simulink model "Proj_5_part_2"  (R2016b)
settings: Solver=ode4  StartTime=0.0  StopTime=1370  FixedStep=0.0001  RelTol=1e-3
undefined symbols (not defined in the file or in its folder): V
settings Model: Creator=apple  LastModifiedBy=apple

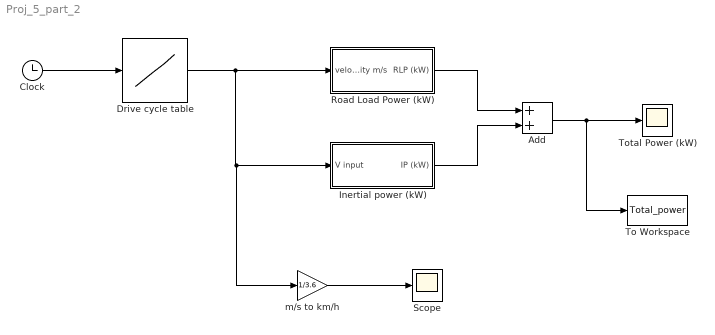
== system Proj_5_part_2 ==
  Add : Sum
  Clock : Clock
  Drive cycle table : Lookup_n-D  NumberOfTableDimensions=1  BreakpointsForDimension1=t  Table=V  InternalRulePriority=Speed  RndMeth=Simplest  InputSameDT=on
  Inertial power (kW) : Subsystem  TreatAsAtomicUnit=on
  Road Load Power (kW) : Subsystem  TreatAsAtomicUnit=on
  Scope : Scope
  To Workspace : ToWorkspace  VariableName=Total_power  SaveFormat=Timeseries  SampleTime=-1
  Total Power (kW) : Scope
  m/s to km/h : Gain  Gain=1/3.6
  wires:
  Clock/1 -> Drive cycle table/1
  Drive cycle table/1 -> m/s to km/h/1, Inertial power (kW)/1(V input), Road Load Power (kW)/1("velocity m/s ")
  Road Load Power (kW)/1(RLP (kW)) -> Add/1
  Inertial power (kW)/1(IP (kW)) -> Add/2
  Add/1 -> To Workspace/1, Total Power (kW)/1
  m/s to km/h/1 -> Scope/1

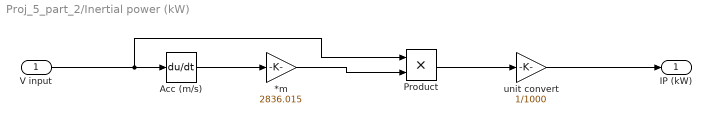
== system Proj_5_part_2/Inertial power (kW) ==
  V input : Inport
  *m : Gain  Gain=2836.015
  Acc (m/s) : Derivative
  Product : Product
  unit convert : Gain  Gain=1/1000
  IP (kW) : Outport
  wires:
  V input/1 -> Product/1, Acc (m/s)/1
  Acc (m/s)/1 -> *m/1
  *m/1 -> Product/2
  Product/1 -> unit convert/1
  unit convert/1 -> IP (kW)/1

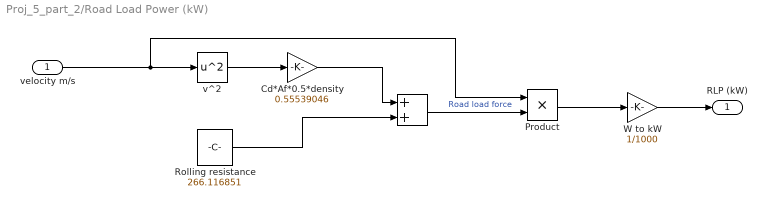
== system Proj_5_part_2/Road Load Power (kW) ==
  "velocity m/s " : Inport
  " " : Sum
  "Cd*Af*0.5*density " : Gain  Gain=0.55539046
  Product : Product
  "Rolling resistance " : Constant  Value=266.116851
  W to kW : Gain  Gain=1/1000
  v^2 : Math  Operator=square  SaturateOnIntegerOverflow=on
  RLP (kW) : Outport
  wires:
  v^2/1 -> "Cd*Af*0.5*density "/1
  "velocity m/s "/1 -> Product/1, v^2/1
  "Cd*Af*0.5*density "/1 -> " "/1
  "Rolling resistance "/1 -> " "/2
  " "/1 -> Product/2  "Road load force"
  Product/1 -> W to kW/1
  W to kW/1 -> RLP (kW)/1
